simulink model "HVAC_HEATER"  (R2018b)
settings: Solver=VariableStepAuto  StartTime=0.0  StopTime=10.0  RelTol=1e-3
settings Model: Creator=Ali Goudarzi  LastModifiedBy=Ali Goudarzi

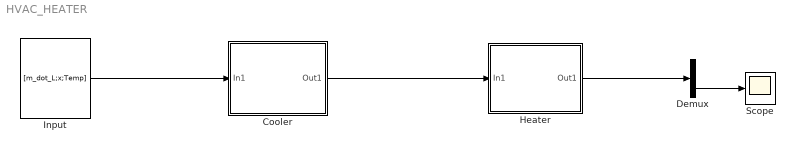
== system HVAC_HEATER ==
  Cooler : Subsystem  mask{Q_dot_cooler=-500}
  Demux : Demux  Outputs=3
  Heater : Subsystem  mask{TempHeater=40}
      mask prompts: TempHeater "Temp Heater"
  Input : Constant  Value=[m_dot_L;x;Temp]  OutDataTypeStr=double  mask{m_dot_L=1, x=0.5, Temp=20}
  Scope : Scope
  wires:
  Heater/1(Out1) -> Demux/1
  Demux/3 -> Scope/1
  Input/1 -> Cooler/1(In1)
  Cooler/1(Out1) -> Heater/1(In1)

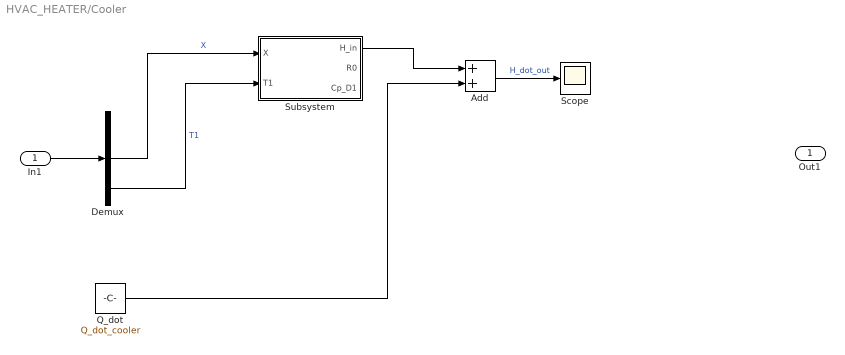
== system HVAC_HEATER/Cooler ==
  In1 : Inport
  Add : Sum
  Demux : Demux  Outputs=3
  Q_dot : Constant  Value=Q_dot_cooler
  Scope : Scope
  Subsystem : Subsystem
  Out1 : Outport
  wires:
  In1/1 -> Demux/1
  Demux/3 -> Subsystem/2(T1)  "T1"
  Demux/2 -> Subsystem/1(X)  "X"
  Subsystem/1(H_in) -> Add/1
  Q_dot/1 -> Add/2
  Add/1 -> Scope/1  "H_dot_out"

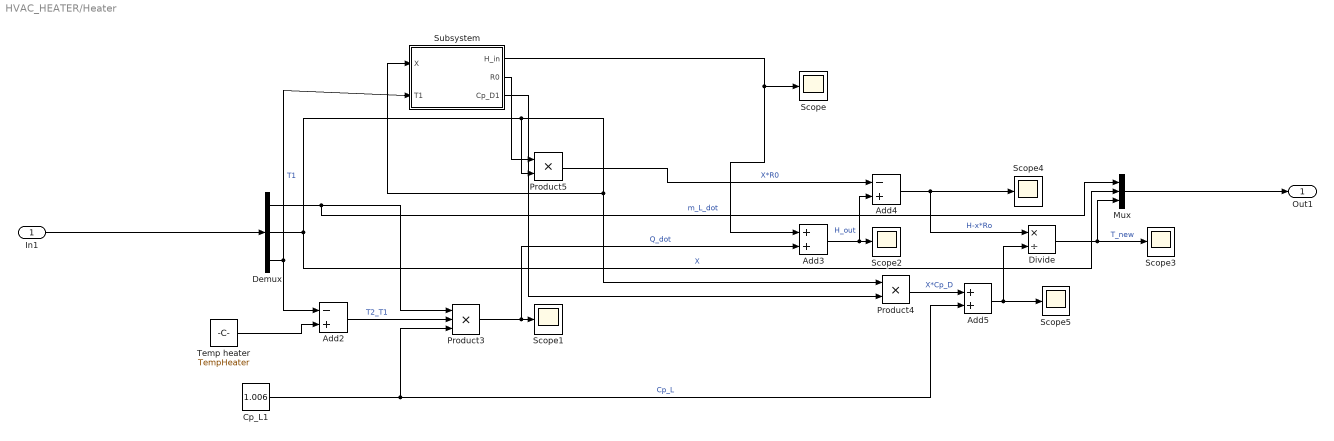
== system HVAC_HEATER/Heater ==
  In1 : Inport
  Add2 : Sum  Inputs=-+
  Add3 : Sum
  Add4 : Sum  Inputs=-+
  Add5 : Sum
  Cp_L1 : Constant  Value=1.006
  Demux : Demux  Outputs=3
  Divide : Product  Inputs=*/
  Mux : Mux  Inputs=3
  Product3 : Product  Inputs=3
  Product4 : Product
  Product5 : Product
  Scope{,1..5} (6 alike) : Scope
  Subsystem : Subsystem
  Temp heater : Constant  Value=TempHeater
  Out1 : Outport
  wires:
  Add4/1 -> Divide/1, Scope4/1  "H-x*Ro"
  Demux/2 -> Mux/2, Product5/2, Subsystem/1(X), Product4/1  "X"
  Add5/1 -> Scope5/1, Divide/2
  Cp_L1/1 -> Add5/2, Product3/3  "Cp_L"
  Product3/1 -> Add3/2, Scope1/1  "Q_dot"
  Add3/1 -> Add4/2, Scope2/1  "H_out"
  Demux/3 -> Subsystem/2(T1), Add2/1  "T1"
  Product4/1 -> Add5/1  "X*Cp_D"
  Add2/1 -> Product3/2  "T2_T1"
  Demux/1 -> Mux/1, Product3/1  "m_L_dot"
  Divide/1 -> Mux/3, Scope3/1  "T_new"
  Product5/1 -> Add4/1  "X*R0"
  In1/1 -> Demux/1
  Mux/1 -> Out1/1
  Temp heater/1 -> Add2/2
  Subsystem/1(H_in) -> Add3/1, Scope/1
  Subsystem/2(R0) -> Product5/1
  Subsystem/3(Cp_D1) -> Product4/2

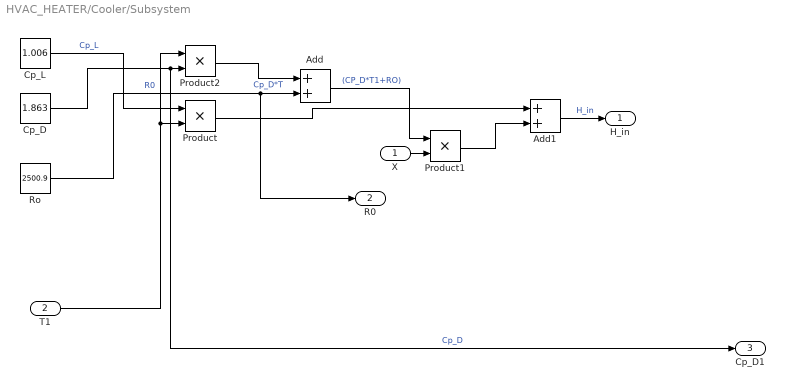
== system HVAC_HEATER/Cooler/Subsystem ==
  X : Inport
  T1 : Inport  Port=2
  Add : Sum
  Add1 : Sum
  Cp_D : Constant  Value=1.863
  Cp_L : Constant  Value=1.006
  Product : Product
  Product1 : Product
  Product2 : Product
  Ro : Constant  Value=2500.9
  H_in : Outport
  R0 : Outport  Port=2
  Cp_D1 : Outport  Port=3
  wires:
  Product/1 -> Add1/1
  Cp_D/1 -> Cp_D1/1, Product2/2  "Cp_D"
  Product1/1 -> Add1/2
  X/1 -> Product1/2
  Ro/1 -> R0/1, Add/2  "R0"
  Product2/1 -> Add/1  "Cp_D*T"
  Add/1 -> Product1/1  "(CP_D*T1+RO)"
  T1/1 -> Product/2, Product2/1
  Cp_L/1 -> Product/1  "Cp_L"
  Add1/1 -> H_in/1  "H_in"

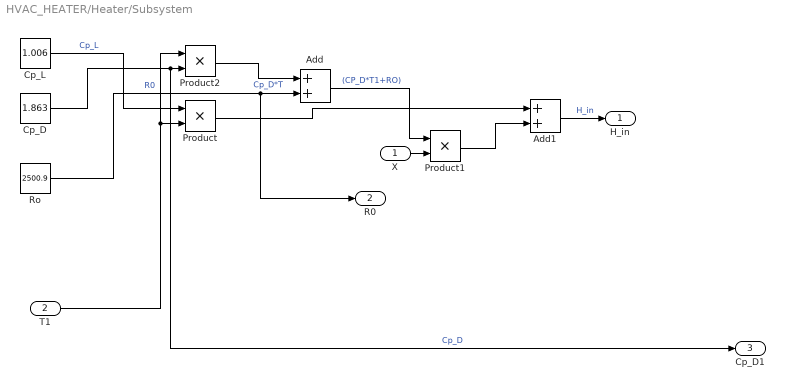
== system HVAC_HEATER/Heater/Subsystem ==
  X : Inport
  T1 : Inport  Port=2
  Add : Sum
  Add1 : Sum
  Cp_D : Constant  Value=1.863
  Cp_L : Constant  Value=1.006
  Product : Product
  Product1 : Product
  Product2 : Product
  Ro : Constant  Value=2500.9
  H_in : Outport
  R0 : Outport  Port=2
  Cp_D1 : Outport  Port=3
  wires:
  Product/1 -> Add1/1
  Cp_D/1 -> Cp_D1/1, Product2/2  "Cp_D"
  Product1/1 -> Add1/2
  X/1 -> Product1/2
  Ro/1 -> R0/1, Add/2  "R0"
  Product2/1 -> Add/1  "Cp_D*T"
  Add/1 -> Product1/1  "(CP_D*T1+RO)"
  T1/1 -> Product/2, Product2/1
  Cp_L/1 -> Product/1  "Cp_L"
  Add1/1 -> H_in/1  "H_in"
